simulink model "SFF_Simulator"  (R2024a)
settings: Solver=FixedStepAuto  StartTime=0.0  StopTime=tf  FixedStep=step_modelo  RelTol=1e-3
values from neighbouring files (symbols this model uses):
  AttKd_x = inp(4,2).Var2    [SFF_Simulator_Entradas.m]
  AttKd_y = inp(5,2).Var2    [SFF_Simulator_Entradas.m]
  AttKd_z = inp(6,2).Var2    [SFF_Simulator_Entradas.m]
  AttKp_x = inp(1,2).Var2    [SFF_Simulator_Entradas.m]
  AttKp_y = inp(2,2).Var2    [SFF_Simulator_Entradas.m]
  AttKp_z = inp(3,2).Var2    [SFF_Simulator_Entradas.m]
  beta = inp(2,2).Var2    [SFF_Simulator_Entradas.m]
  cdgps = inp(1,2).Var2    [SFF_Simulator_Entradas.m]
  estrelas = inp(4,2).Var2    [SFF_Simulator_Entradas.m]
  estrelas_bias = inp(6,2).Var2    [SFF_Simulator_Entradas.m]
  estrelas_ruido = inp(5,2).Var2    [SFF_Simulator_Entradas.m]
  gps_bias = inp(3,2).Var2    [SFF_Simulator_Entradas.m]
  gps_ruido = inp(2,2).Var2    [SFF_Simulator_Entradas.m]
  m1 = inp(6,2).Var2    [SFF_Simulator_Entradas.m]
  magne = inp(10,2).Var2    [SFF_Simulator_Entradas.m]
  magne_bias = inp(12,2).Var2    [SFF_Simulator_Entradas.m]
  magne_ruido = inp(11,2).Var2    [SFF_Simulator_Entradas.m]
  man = inp(1,2).Var2    [SFF_Simulator_Entradas.m]
  OrbKd_x = inp(3,2).Var2    [SFF_Simulator_Entradas.m]
  OrbKd_y = inp(6,2).Var2    [SFF_Simulator_Entradas.m]
  OrbKd_z = inp(9,2).Var2    [SFF_Simulator_Entradas.m]
  OrbKi_x = inp(2,2).Var2    [SFF_Simulator_Entradas.m]
  OrbKi_y = inp(5,2).Var2    [SFF_Simulator_Entradas.m]
  OrbKi_z = inp(8,2).Var2    [SFF_Simulator_Entradas.m]
  OrbKp_x = inp(1,2).Var2    [SFF_Simulator_Entradas.m]
  OrbKp_y = inp(4,2).Var2    [SFF_Simulator_Entradas.m]
  OrbKp_z = inp(7,2).Var2    [SFF_Simulator_Entradas.m]
  propForcaAtivo = inp(1,2).Var2    [SFF_Simulator_Entradas.m]
  rodaAtivo = inp(1,2).Var2    [SFF_Simulator_Entradas.m]
  torqrodAtivo = inp(1,2).Var2    [SFF_Simulator_Entradas.m]
undefined symbols (not defined in the file or in its folder): IAU, WMM2020
libraries: dspsrcs4 x9, aerolibtransform2 x1, aerolibgravity2 x1
(part 1 of 2)
settings Model: PacingRate=1000  VariantFading=off  Creator=rodri  LastModifiedBy=rodri
settings ModelReferenceCC: ModelReferenceMinAlgLoopOccurrences=on
settings RTWCC: GPUComputeCapability=3.5

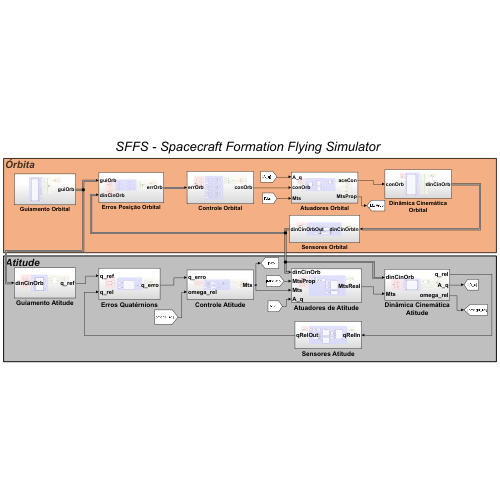
[thumbnail: Simulink's stored preview of the top-level diagram]
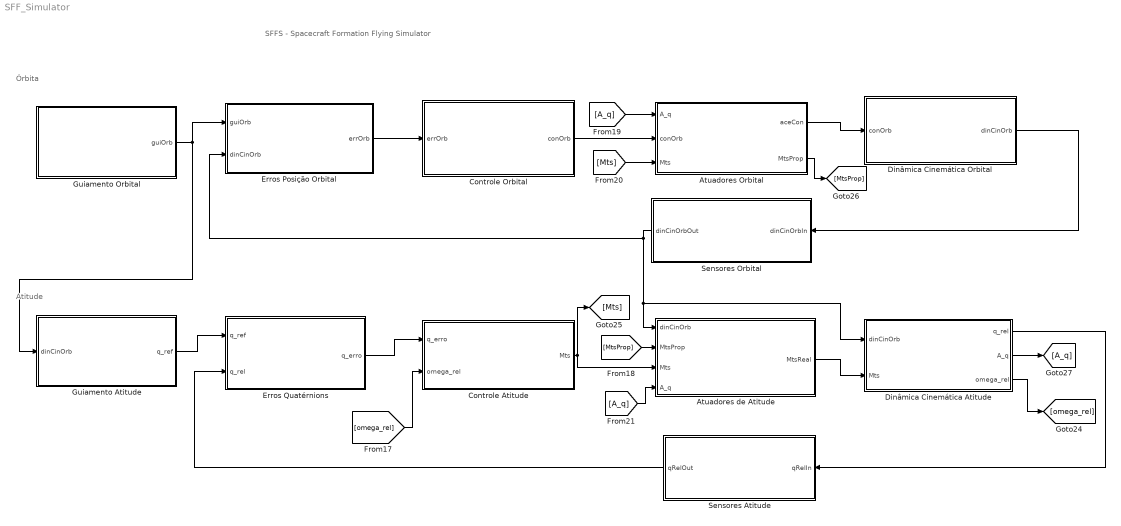
== system SFF_Simulator ==
  note: SFFS - Spacecraft Formation Flying Simulator
  note: Atitude
  note: Órbita
  Atuadores Orbital : Subsystem
  Atuadores de Atitude : Subsystem
  Controle Atitude : Subsystem
  Controle Orbital : Subsystem
  Dinâmica Cinemática Atitude : Subsystem
  Dinâmica Cinemática Orbital : Subsystem
  Erros Posição Orbital : Subsystem
  Erros Quatérnions : Subsystem
  Guiamento Atitude : Subsystem
  Guiamento Orbital : Subsystem
  Sensores Atitude : Subsystem
  Sensores Orbital : Subsystem
  wires:
  [omega_rel] -> Controle Atitude/2(omega_rel)
  Erros Quatérnions/1(q_erro) -> Controle Atitude/1(q_erro)
  Dinâmica Cinemática Atitude/2(A_q) -> [A_q]
  [A_q] -> Atuadores Orbital/1(A_q)
  Atuadores Orbital/1(aceCon) -> Dinâmica Cinemática Orbital/1(conOrb)
  Erros Posição Orbital/1(errOrb) -> Controle Orbital/1(errOrb)
  Dinâmica Cinemática Atitude/1(q_rel) -> Sensores Atitude/1(qRelIn)
  Guiamento Orbital/1(guiOrb) -> Guiamento Atitude/1(dinCinOrb), Erros Posição Orbital/1(guiOrb)
  Dinâmica Cinemática Atitude/3(omega_rel) -> [omega_rel]
  Guiamento Atitude/1(q_ref) -> Erros Quatérnions/1(q_ref)
  [MtsProp] -> Atuadores de Atitude/2(MtsProp)
  [Mts] -> Atuadores Orbital/3(Mts)
  [A_q] -> Atuadores de Atitude/4(A_q)
  Controle Atitude/1(Mts) -> Atuadores de Atitude/3(Mts), [Mts]
  Atuadores de Atitude/1(MtsReal) -> Dinâmica Cinemática Atitude/2(Mts)
  Atuadores Orbital/2(MtsProp) -> [MtsProp]
  Sensores Orbital/1(dinCinOrbOut) -> Dinâmica Cinemática Atitude/1(dinCinOrb), Atuadores de Atitude/1(dinCinOrb), Erros Posição Orbital/2(dinCinOrb)
  Controle Orbital/1(conOrb) -> Atuadores Orbital/2(conOrb)
  Sensores Atitude/1(qRelOut) -> Erros Quatérnions/2(q_rel)
  Dinâmica Cinemática Orbital/1(dinCinOrb) -> Sensores Orbital/1(dinCinOrbIn)

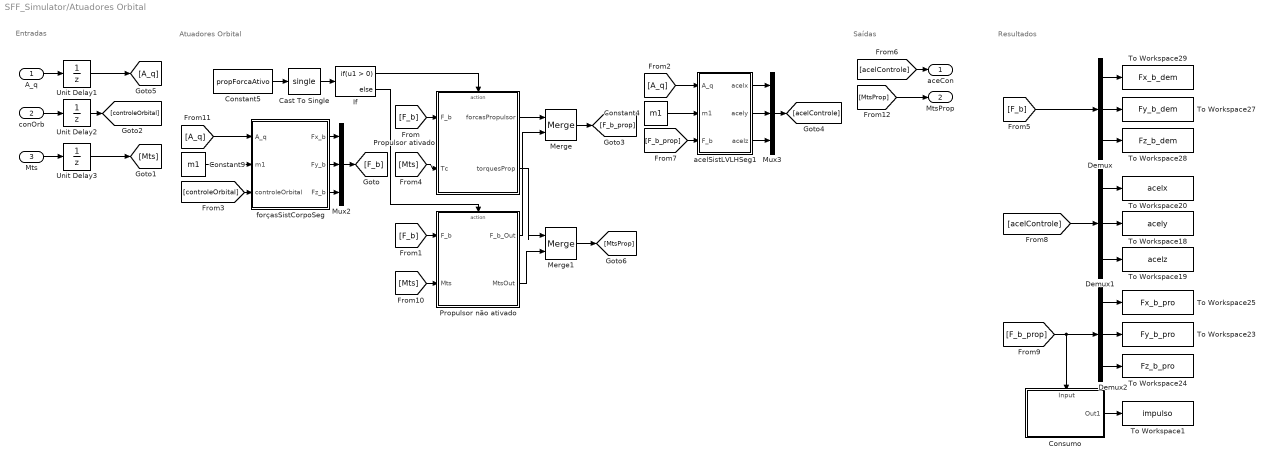
== system SFF_Simulator/Atuadores Orbital ==
  note: Resultados
  note: Entradas
  note: Saídas
  note: Atuadores Orbital
  A_q : Inport
  conOrb : Inport  Port=2
  Mts : Inport  Port=3
  Cast To Single : DataTypeConversion  OutDataTypeStr=single  SaturateOnIntegerOverflow=off  RndMeth=Floor
  Constant4 : Constant  Value=m1  SampleTime=-1
  Constant5 : Constant  Value=propForcaAtivo  SampleTime=-1
  Constant9 : Constant  Value=m1  SampleTime=-1
  Consumo : Subsystem
      settings: PortSchema="{\"entries\":[{\"content\":{\"sides\":[{\"content\":{},\"type\":\"ConnectorPlacement.EquallySpacedRectSide\",\"uuid\":\"7adfb598-cfd3-455e-a32c-0f282c9a4562\"},{\"content\":{\"connectorIds\":[\"Out1\"],\"side\":\"RIGHT\"},\"type\":\"ConnectorPlacement.EquallySpacedRectSide\",\"uuid\":\"983f0880-1b1d-4863-83b8-6f46272dfc63\"},{\"content\":{\"connectorIds\":[\"In1\"],\"side\":\"TOP\"},\"type\":\"ConnectorPlacement.EquallySpacedRectSide\",\"uuid\":\"1e4b7baa-07be-492c-ad2b-c1f0c72f4a8d\"}]},\"type\":\"ConnectorPlacement.EquallySpacedConnector\",\"uuid\":\"1ca021a5-bfd9-4f0e-bb93-1261a452b994\"}],\"packageUris\":[\"http://schema.mathworks.com/mf0/Connector/R2020b\"],\"version\":\"1.0\"}"
  Demux : Demux  Outputs=3
  Demux1 : Demux  Outputs=3
  Demux2 : Demux  Outputs=3
  If : If
  Merge : Merge
  Merge1 : Merge
  Mux2 : Mux  Inputs=3
  Mux3 : Mux  Inputs=3
  Propulsor ativado : Subsystem  TreatAsAtomicUnit=on
  Propulsor não ativado : Subsystem  TreatAsAtomicUnit=on
  To Workspace1 : ToWorkspace  VariableName=impulso  SampleTime=-1
      settings: Save2DSignal=2-D array (concatenate along first dimension)
  To Workspace18 : ToWorkspace  VariableName=acely  SampleTime=-1
      settings: Save2DSignal=2-D array (concatenate along first dimension)
  To Workspace19 : ToWorkspace  VariableName=acelz  SampleTime=-1
      settings: Save2DSignal=2-D array (concatenate along first dimension)
  To Workspace20 : ToWorkspace  VariableName=acelx  SampleTime=-1
      settings: Save2DSignal=2-D array (concatenate along first dimension)
  To Workspace23 : ToWorkspace  VariableName=Fy_b_pro  SampleTime=-1
      settings: Save2DSignal=2-D array (concatenate along first dimension)
  To Workspace24 : ToWorkspace  VariableName=Fz_b_pro  SampleTime=-1
      settings: Save2DSignal=2-D array (concatenate along first dimension)
  To Workspace25 : ToWorkspace  VariableName=Fx_b_pro  SampleTime=-1
      settings: Save2DSignal=2-D array (concatenate along first dimension)
  To Workspace27 : ToWorkspace  VariableName=Fy_b_dem  SampleTime=-1
      settings: Save2DSignal=2-D array (concatenate along first dimension)
  To Workspace28 : ToWorkspace  VariableName=Fz_b_dem  SampleTime=-1
      settings: Save2DSignal=2-D array (concatenate along first dimension)
  To Workspace29 : ToWorkspace  VariableName=Fx_b_dem  SampleTime=-1
      settings: Save2DSignal=2-D array (concatenate along first dimension)
  Unit Delay1 : UnitDelay  SampleTime=-1  HasFrameUpgradeWarning=on
  Unit Delay2 : UnitDelay  SampleTime=-1  HasFrameUpgradeWarning=on
  Unit Delay3 : UnitDelay  SampleTime=-1  HasFrameUpgradeWarning=on
  acelSistLVLHSeg1 : MATLAB Function  TreatAsAtomicUnit=on
  forçasSistCorpoSeg : MATLAB Function  TreatAsAtomicUnit=on
  aceCon : Outport
  MtsProp : Outport  Port=2
  wires:
  Demux1/3 -> To Workspace19/1
  Demux1/1 -> To Workspace20/1
  Demux1/2 -> To Workspace18/1
  [acelControle] -> Demux1/1
  Consumo/1(Out1) -> To Workspace1/1
  Demux/1 -> To Workspace29/1
  Demux/2 -> To Workspace27/1
  Demux/3 -> To Workspace28/1
  [F_b] -> Demux/1
  Demux2/1 -> To Workspace25/1
  [F_b_prop] -> Demux2/1, Consumo/1(Input)
  Demux2/2 -> To Workspace23/1
  Demux2/3 -> To Workspace24/1
  [A_q] -> acelSistLVLHSeg1/1(A_q)
  [acelControle] -> aceCon/1
  [F_b_prop] -> acelSistLVLHSeg1/3(F_b)
  [MtsProp] -> MtsProp/1
  Constant4/1 -> acelSistLVLHSeg1/2(m1)
  Propulsor ativado/2(torquesProp) -> Merge1/1
  Merge/1 -> [F_b_prop]
  forçasSistCorpoSeg/3(Fz_b) -> Mux2/3
  Unit Delay1/1 -> [A_q]
  Merge1/1 -> [MtsProp]
  forçasSistCorpoSeg/1(Fx_b) -> Mux2/1
  If/2 -> Propulsor não ativado/Action
  If/1 -> Propulsor ativado/Action
  Unit Delay2/1 -> [controleOrbital]
  [Mts] -> Propulsor não ativado/2(Mts)
  [A_q] -> forçasSistCorpoSeg/1(A_q)
  Constant9/1 -> forçasSistCorpoSeg/2(m1)
  [controleOrbital] -> forçasSistCorpoSeg/3(controleOrbital)
  [Mts] -> Propulsor ativado/2(Tc)
  acelSistLVLHSeg1/1(acelx) -> Mux3/1
  Mux3/1 -> [acelControle]
  acelSistLVLHSeg1/3(acelz) -> Mux3/3
  acelSistLVLHSeg1/2(acely) -> Mux3/2
  forçasSistCorpoSeg/2(Fy_b) -> Mux2/2
  Propulsor ativado/1(forcasPropulsor) -> Merge/1
  Cast To Single/1 -> If/1
  Mux2/1 -> [F_b]
  Mts/1 -> Unit Delay3/1
  [F_b] -> Propulsor não ativado/1(F_b)
  conOrb/1 -> Unit Delay2/1
  Propulsor não ativado/1(F_b_Out) -> Merge/2
  Unit Delay3/1 -> [Mts]
  Constant5/1 -> Cast To Single/1
  [F_b] -> Propulsor ativado/1(F_b)
  Propulsor não ativado/2(MtsOut) -> Merge1/2
  A_q/1 -> Unit Delay1/1

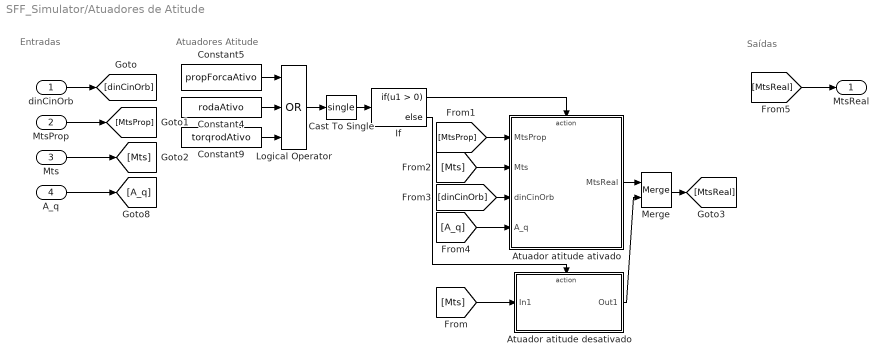
== system SFF_Simulator/Atuadores de Atitude ==
  note: Entradas
  note: Atuadores Atitude
  note: Saídas
  dinCinOrb : Inport
  MtsProp : Inport  Port=2
  Mts : Inport  Port=3
  A_q : Inport  Port=4
  Atuador atitude ativado : Subsystem  TreatAsAtomicUnit=on
  Atuador atitude desativado : Subsystem  TreatAsAtomicUnit=on
  Cast To Single : DataTypeConversion  OutDataTypeStr=single  SaturateOnIntegerOverflow=off  RndMeth=Floor
  Constant4 : Constant  Value=rodaAtivo  SampleTime=-1
  Constant5 : Constant  Value=propForcaAtivo  SampleTime=-1
  Constant9 : Constant  Value=torqrodAtivo  SampleTime=-1
  If : If
  Logical Operator : Logic  Operator=OR  Inputs=3  AllPortsSameDT=off  OutDataTypeStr=boolean
  Merge : Merge
  MtsReal : Outport
  wires:
  Mts/1 -> [Mts]
  dinCinOrb/1 -> [dinCinOrb]
  MtsProp/1 -> [MtsProp]
  Merge/1 -> [MtsReal]
  If/1 -> Atuador atitude ativado/Action
  If/2 -> Atuador atitude desativado/Action
  Atuador atitude ativado/1(MtsReal) -> Merge/1
  Atuador atitude desativado/1(Out1) -> Merge/2
  [Mts] -> Atuador atitude desativado/1(In1)
  [MtsProp] -> Atuador atitude ativado/1(MtsProp)
  [Mts] -> Atuador atitude ativado/2(Mts)
  [dinCinOrb] -> Atuador atitude ativado/3(dinCinOrb)
  [A_q] -> Atuador atitude ativado/4(A_q)
  A_q/1 -> [A_q]
  [MtsReal] -> MtsReal/1
  Constant5/1 -> Logical Operator/1
  Logical Operator/1 -> Cast To Single/1
  Cast To Single/1 -> If/1
  Constant4/1 -> Logical Operator/2
  Constant9/1 -> Logical Operator/3

== system SFF_Simulator/Controle Atitude ==
  note: Entradas
  note: Controle de Atitude
  note: Saídas
  note: Resultados
  q_erro : Inport
  omega_rel : Inport  Port=2
  Demux : Demux
  Demux1 : Demux  Outputs=3
  Demux3 : Demux  Outputs=3
  Gain1 : Gain  Gain=-1
  Kd1 : Gain  Gain=[AttKd_x AttKd_y AttKd_z]'
  Kp1 : Gain  Gain=[AttKp_x AttKp_y AttKp_z]'
  Mux : Mux  Inputs=3
  Sum3 : Sum  Inputs=|++
  Terminator : Terminator
  To Workspace24 : ToWorkspace  VariableName=Mts_x  SampleTime=-1
      settings: Save2DSignal=2-D array (concatenate along first dimension)
  To Workspace25 : ToWorkspace  VariableName=Mts_y  SampleTime=-1
      settings: Save2DSignal=2-D array (concatenate along first dimension)
  To Workspace26 : ToWorkspace  VariableName=Mts_z  SampleTime=-1
      settings: Save2DSignal=2-D array (concatenate along first dimension)
  Unit Delay : UnitDelay  SampleTime=-1  HasFrameUpgradeWarning=on
  Unit Delay1 : UnitDelay  SampleTime=-1  HasFrameUpgradeWarning=on
  Vector Concatenate1 : Concatenate  NumInputs=3  Mode=Multidimensional array
  Mts : Outport
  wires:
  [q_erro] -> Demux/1
  Mux/1 -> Kp1/1
  Demux/1 -> Mux/1
  Demux/2 -> Mux/2
  Demux/3 -> Mux/3
  Demux/4 -> Terminator/1
  [omega_rel] -> Kd1/1
  Kd1/1 -> Sum3/2
  Sum3/1 -> Demux1/1
  Demux1/1 -> Vector Concatenate1/1
  Demux1/2 -> Vector Concatenate1/2
  Demux1/3 -> Vector Concatenate1/3
  q_erro/1 -> Unit Delay/1
  omega_rel/1 -> Unit Delay1/1
  [Mts] -> Mts/1
  Vector Concatenate1/1 -> Gain1/1
  Gain1/1 -> [Mts]
  Kp1/1 -> Sum3/1
  Demux3/3 -> To Workspace26/1
  Demux3/2 -> To Workspace25/1
  Demux3/1 -> To Workspace24/1
  [Mts] -> Demux3/1
  Unit Delay/1 -> [q_erro]
  Unit Delay1/1 -> [omega_rel]

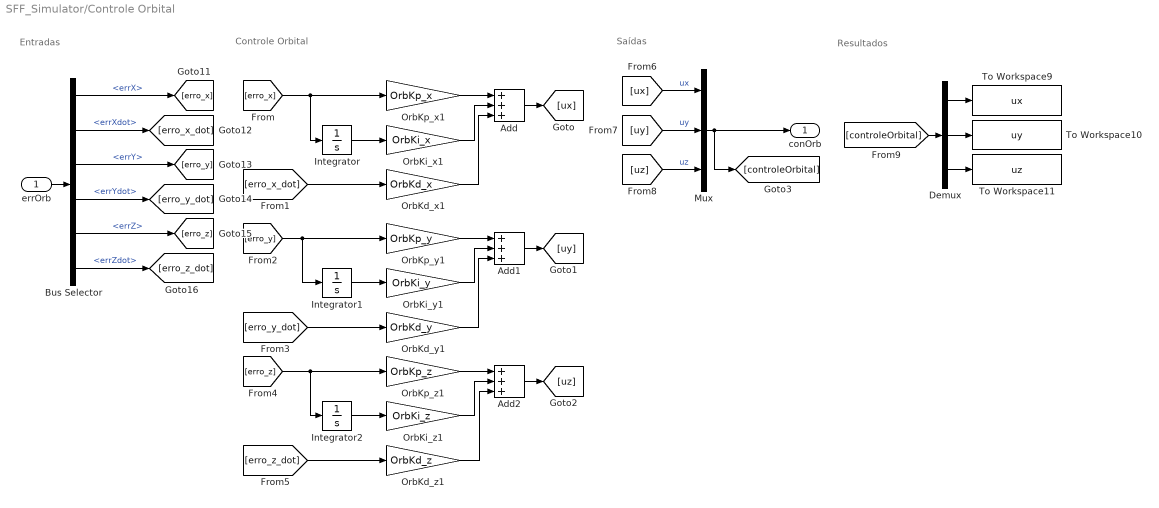
== system SFF_Simulator/Controle Orbital ==
  note: Entradas
  note: Controle Orbital
  note: Saídas
  note: Resultados
  errOrb : Inport
  Add : Sum  Inputs=+++
  Add1 : Sum  Inputs=+++
  Add2 : Sum  Inputs=+++
  Bus Selector : BusSelector  OutputSignals=errX,errXdot,errY,errYdot,errZ,errZdot
  Demux : Demux  Outputs=3
  Integrator : Integrator
  Integrator1 : Integrator
  Integrator2 : Integrator
  Mux : Mux  Inputs=3
  OrbKd_x1 : Gain  Gain=OrbKd_x
  OrbKd_y1 : Gain  Gain=OrbKd_y
  OrbKd_z1 : Gain  Gain=OrbKd_z
  OrbKi_x1 : Gain  Gain=OrbKi_x
  OrbKi_y1 : Gain  Gain=OrbKi_y
  OrbKi_z1 : Gain  Gain=OrbKi_z
  OrbKp_x1 : Gain  Gain=OrbKp_x
  OrbKp_y1 : Gain  Gain=OrbKp_y
  OrbKp_z1 : Gain  Gain=OrbKp_z
  To Workspace10 : ToWorkspace  VariableName=uy  SampleTime=-1
      settings: Save2DSignal=2-D array (concatenate along first dimension)
  To Workspace11 : ToWorkspace  VariableName=uz  SampleTime=-1
      settings: Save2DSignal=2-D array (concatenate along first dimension)
  To Workspace9 : ToWorkspace  VariableName=ux  SampleTime=-1
      settings: Save2DSignal=2-D array (concatenate along first dimension)
  conOrb : Outport
  wires:
  Add/1 -> [ux]
  Add1/1 -> [uy]
  Add2/1 -> [uz]
  Bus Selector/6 -> [erro_z_dot]  "<errZdot>"
  Bus Selector/4 -> [erro_y_dot]  "<errYdot>"
  Bus Selector/3 -> [erro_y]  "<errY>"
  Bus Selector/1 -> [erro_x]  "<errX>"
  Bus Selector/5 -> [erro_z]  "<errZ>"
  Bus Selector/2 -> [erro_x_dot]  "<errXdot>"
  errOrb/1 -> Bus Selector/1
  [ux] -> Mux/1  "ux"
  [uy] -> Mux/2  "uy"
  [uz] -> Mux/3  "uz"
  [erro_x_dot] -> OrbKd_x1/1
  Integrator1/1 -> OrbKi_y1/1
  Integrator2/1 -> OrbKi_z1/1
  [erro_y] -> OrbKp_y1/1, Integrator1/1
  OrbKi_z1/1 -> Add2/2
  OrbKi_x1/1 -> Add/2
  OrbKp_x1/1 -> Add/1
  OrbKd_x1/1 -> Add/3
  [erro_x] -> OrbKp_x1/1, Integrator/1
  OrbKi_y1/1 -> Add1/2
  OrbKp_y1/1 -> Add1/1
  Integrator/1 -> OrbKi_x1/1
  OrbKd_y1/1 -> Add1/3
  [erro_z_dot] -> OrbKd_z1/1
  OrbKd_z1/1 -> Add2/3
  [erro_y_dot] -> OrbKd_y1/1
  [erro_z] -> OrbKp_z1/1, Integrator2/1
  OrbKp_z1/1 -> Add2/1
  Mux/1 -> conOrb/1, [controleOrbital]
  Demux/3 -> To Workspace11/1
  [controleOrbital] -> Demux/1
  Demux/1 -> To Workspace9/1
  Demux/2 -> To Workspace10/1

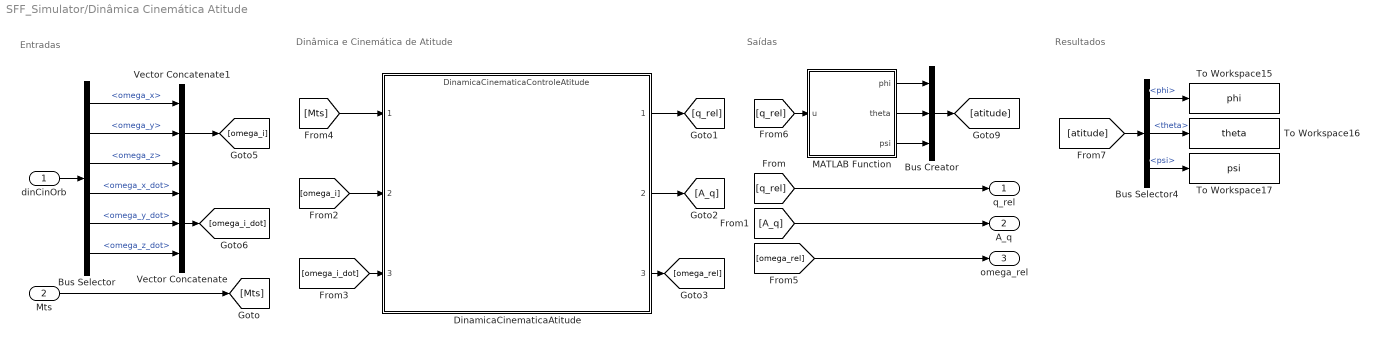
== system SFF_Simulator/Dinâmica Cinemática Atitude ==
  note: Dinâmica e Cinemática de Atitude
  note: Saídas
  note: Entradas
  note: Resultados
  dinCinOrb : Inport
  Mts : Inport  Port=2
  Bus Creator : BusCreator  Inputs=3
  Bus Selector : BusSelector  OutputSignals=omega_x,omega_y,omega_z,omega_x_dot,omega_y_dot,omega_z_dot
  Bus Selector4 : BusSelector  OutputSignals=phi,theta,psi
  DinamicaCinematicaAtitude : ModelReference  ModelNameDialog=DinamicaCinematicaControleAtitude  ModelReferenceVersion=3.15
  MATLAB Function : MATLAB Function  TreatAsAtomicUnit=on
  To Workspace15 : ToWorkspace  VariableName=phi  SampleTime=-1
      settings: Save2DSignal=2-D array (concatenate along first dimension)
  To Workspace16 : ToWorkspace  VariableName=theta  SampleTime=-1
      settings: Save2DSignal=2-D array (concatenate along first dimension)
  To Workspace17 : ToWorkspace  VariableName=psi  SampleTime=-1
      settings: Save2DSignal=2-D array (concatenate along first dimension)
  Vector Concatenate : Concatenate  NumInputs=3  Mode=Multidimensional array
  Vector Concatenate1 : Concatenate  NumInputs=3  Mode=Multidimensional array
  q_rel : Outport
  A_q : Outport  Port=2
  omega_rel : Outport  Port=3
  wires:
  DinamicaCinematicaAtitude/1 -> [q_rel]
  DinamicaCinematicaAtitude/2 -> [A_q]
  [q_rel] -> q_rel/1
  dinCinOrb/1 -> Bus Selector/1
  [omega_i] -> DinamicaCinematicaAtitude/2
  [omega_i_dot] -> DinamicaCinematicaAtitude/3
  [Mts] -> DinamicaCinematicaAtitude/1
  Bus Selector/1 -> Vector Concatenate1/1  "<omega_x>"
  Bus Selector/3 -> Vector Concatenate1/3  "<omega_z>"
  Bus Selector/2 -> Vector Concatenate1/2  "<omega_y>"
  Vector Concatenate1/1 -> [omega_i]
  Bus Selector/4 -> Vector Concatenate/1  "<omega_x_dot>"
  Bus Selector/5 -> Vector Concatenate/2  "<omega_y_dot>"
  Bus Selector/6 -> Vector Concatenate/3  "<omega_z_dot>"
  Vector Concatenate/1 -> [omega_i_dot]
  DinamicaCinematicaAtitude/3 -> [omega_rel]
  Mts/1 -> [Mts]
  [q_rel] -> MATLAB Function/1(u)
  MATLAB Function/1(phi) -> Bus Creator/1
  MATLAB Function/2(theta) -> Bus Creator/2
  MATLAB Function/3(psi) -> Bus Creator/3
  [A_q] -> A_q/1
  [omega_rel] -> omega_rel/1
  Bus Selector4/2 -> To Workspace16/1  "<theta>"
  Bus Selector4/1 -> To Workspace15/1  "<phi>"
  [atitude] -> Bus Selector4/1
  Bus Selector4/3 -> To Workspace17/1  "<psi>"
  Bus Creator/1 -> [atitude]

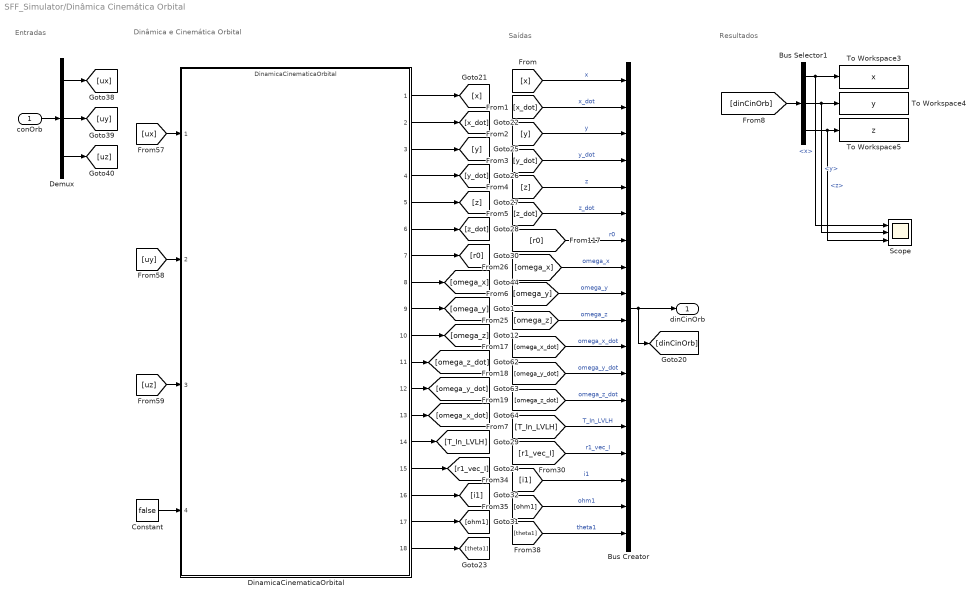
== system SFF_Simulator/Dinâmica Cinemática Orbital ==
  note: Entradas
  note: Saídas
  note: Dinâmica e Cinemática Orbital
  note: Resultados
  conOrb : Inport  OutDataTypeStr=double
  Bus Creator : BusCreator  Inputs=18
  Bus Selector1 : BusSelector  OutputSignals=x,y,z
  Constant : Constant  Value=false
  Demux : Demux  Outputs=3
  DinamicaCinematicaOrbital : ModelReference  ModelNameDialog=DinamicaCinematicaOrbital  ModelReferenceVersion=5.21
  Scope : Scope  NumInputPorts=3
  To Workspace3 : ToWorkspace  VariableName=x  SampleTime=-1
      settings: Save2DSignal=2-D array (concatenate along first dimension)
  To Workspace4 : ToWorkspace  VariableName=y  SampleTime=-1
      settings: Save2DSignal=2-D array (concatenate along first dimension)
  To Workspace5 : ToWorkspace  VariableName=z  SampleTime=-1
      settings: Save2DSignal=2-D array (concatenate along first dimension)
  dinCinOrb : Outport
  wires:
  conOrb/1 -> Demux/1
  Demux/1 -> [ux]
  Demux/2 -> [uy]
  Demux/3 -> [uz]
  [ux] -> DinamicaCinematicaOrbital/1
  [uy] -> DinamicaCinematicaOrbital/2
  [uz] -> DinamicaCinematicaOrbital/3
  Constant/1 -> DinamicaCinematicaOrbital/4
  Bus Creator/1 -> dinCinOrb/1, [dinCinOrb]
  Bus Selector1/1 -> To Workspace3/1, Scope/1  "<x>"
  Bus Selector1/2 -> To Workspace4/1, Scope/2  "<y>"
  Bus Selector1/3 -> Scope/3, To Workspace5/1  "<z>"
  [dinCinOrb] -> Bus Selector1/1
  DinamicaCinematicaOrbital/2 -> [x_dot]
  DinamicaCinematicaOrbital/5 -> [z]
  DinamicaCinematicaOrbital/4 -> [y_dot]
  DinamicaCinematicaOrbital/6 -> [z_dot]
  DinamicaCinematicaOrbital/7 -> [r0]
  DinamicaCinematicaOrbital/3 -> [y]
  DinamicaCinematicaOrbital/1 -> [x]
  DinamicaCinematicaOrbital/8 -> [omega_x]
  DinamicaCinematicaOrbital/10 -> [omega_z]
  DinamicaCinematicaOrbital/11 -> [omega_z_dot]
  DinamicaCinematicaOrbital/12 -> [omega_y_dot]
  DinamicaCinematicaOrbital/13 -> [omega_x_dot]
  DinamicaCinematicaOrbital/14 -> [T_In_LVLH]
  DinamicaCinematicaOrbital/15 -> [r1_vec_I]
  DinamicaCinematicaOrbital/16 -> [i1]
  DinamicaCinematicaOrbital/17 -> [ohm1]
  DinamicaCinematicaOrbital/18 -> [theta1]
  DinamicaCinematicaOrbital/9 -> [omega_y]
  [theta1] -> Bus Creator/18  "theta1"
  [ohm1] -> Bus Creator/17  "ohm1"
  [i1] -> Bus Creator/16  "i1"
  [r1_vec_I] -> Bus Creator/15  "r1_vec_I"
  [T_In_LVLH] -> Bus Creator/14  "T_In_LVLH"
  [omega_z_dot] -> Bus Creator/13  "omega_z_dot"
  [omega_y_dot] -> Bus Creator/12  "omega_y_dot"
  [omega_x_dot] -> Bus Creator/11  "omega_x_dot"
  [omega_z] -> Bus Creator/10  "omega_z"
  [omega_y] -> Bus Creator/9  "omega_y"
  [omega_x] -> Bus Creator/8  "omega_x"
  [r0] -> Bus Creator/7  "r0"
  [z_dot] -> Bus Creator/6  "z_dot"
  [z] -> Bus Creator/5  "z"
  [y_dot] -> Bus Creator/4  "y_dot"
  [y] -> Bus Creator/3  "y"
  [x_dot] -> Bus Creator/2  "x_dot"
  [x] -> Bus Creator/1  "x"

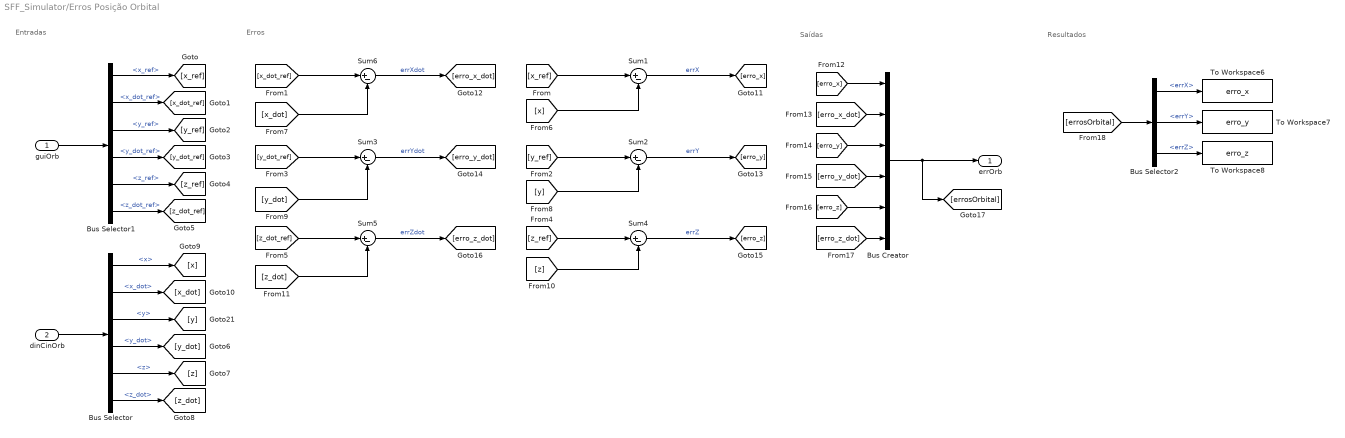
== system SFF_Simulator/Erros Posição Orbital ==
  note: Saídas
  note: Erros
  note: Entradas
  note: Resultados
  guiOrb : Inport
  dinCinOrb : Inport  Port=2
  Bus Creator : BusCreator  Inputs=6
  Bus Selector : BusSelector  OutputSignals=x,x_dot,y,y_dot,z,z_dot
  Bus Selector1 : BusSelector  OutputSignals=x_ref,x_dot_ref,y_ref,y_dot_ref,z_ref,z_dot_ref
  Bus Selector2 : BusSelector  OutputSignals=errX,errY,errZ
  Sum{1..6} (6 alike) : Sum  Inputs=|+-
  To Workspace6 : ToWorkspace  VariableName=erro_x  SampleTime=-1
      settings: Save2DSignal=2-D array (concatenate along first dimension)
  To Workspace7 : ToWorkspace  VariableName=erro_y  SampleTime=-1
      settings: Save2DSignal=2-D array (concatenate along first dimension)
  To Workspace8 : ToWorkspace  VariableName=erro_z  SampleTime=-1
      settings: Save2DSignal=2-D array (concatenate along first dimension)
  errOrb : Outport
  wires:
  [x] -> Sum1/2
  [x_dot] -> Sum6/2
  [x_dot_ref] -> Sum6/1
  [x_ref] -> Sum1/1
  Sum6/1 -> [erro_x_dot]  "errXdot"
  Sum1/1 -> [erro_x]  "errX"
  Sum3/1 -> [erro_y_dot]  "errYdot"
  Sum2/1 -> [erro_y]  "errY"
  [y] -> Sum2/2
  [y_dot] -> Sum3/2
  [y_ref] -> Sum2/1
  [y_dot_ref] -> Sum3/1
  Sum5/1 -> [erro_z_dot]  "errZdot"
  Sum4/1 -> [erro_z]  "errZ"
  [z_dot] -> Sum5/2
  [z_dot_ref] -> Sum5/1
  [z] -> Sum4/2
  [z_ref] -> Sum4/1
  Bus Selector1/4 -> [y_dot_ref]  "<y_dot_ref>"
  Bus Selector1/2 -> [x_dot_ref]  "<x_dot_ref>"
  guiOrb/1 -> Bus Selector1/1
  Bus Selector1/6 -> [z_dot_ref]  "<z_dot_ref>"
  Bus Selector1/3 -> [y_ref]  "<y_ref>"
  Bus Selector1/1 -> [x_ref]  "<x_ref>"
  Bus Selector1/5 -> [z_ref]  "<z_ref>"
  Bus Selector/1 -> [x]  "<x>"
  Bus Selector/4 -> [y_dot]  "<y_dot>"
  Bus Selector/3 -> [y]  "<y>"
  Bus Selector/6 -> [z_dot]  "<z_dot>"
  Bus Selector/5 -> [z]  "<z>"
  Bus Selector/2 -> [x_dot]  "<x_dot>"
  dinCinOrb/1 -> Bus Selector/1
  [erro_x] -> Bus Creator/1
  [erro_x_dot] -> Bus Creator/2
  [erro_y] -> Bus Creator/3
  [erro_y_dot] -> Bus Creator/4
  [erro_z] -> Bus Creator/5
  [erro_z_dot] -> Bus Creator/6
  Bus Selector2/2 -> To Workspace7/1  "<errY>"
  Bus Selector2/3 -> To Workspace8/1  "<errZ>"
  Bus Selector2/1 -> To Workspace6/1  "<errX>"
  [errosOrbital] -> Bus Selector2/1
  Bus Creator/1 -> [errosOrbital], errOrb/1

== system SFF_Simulator/Erros Quatérnions ==
  note: Erros
  note: Saídas
  note: Entradas
  q_ref : Inport
  q_rel : Inport  Port=2
  MATLAB Function4 : MATLAB Function  TreatAsAtomicUnit=on
  q_erro : Outport
  wires:
  [q_ref] -> MATLAB Function4/1(q_d)
  [q_rel] -> MATLAB Function4/2(q)
  MATLAB Function4/1(q_error) -> [q_erro]  "q_erro"
  [q_erro] -> q_erro/1
  q_rel/1 -> [q_rel]
  q_ref/1 -> [q_ref]

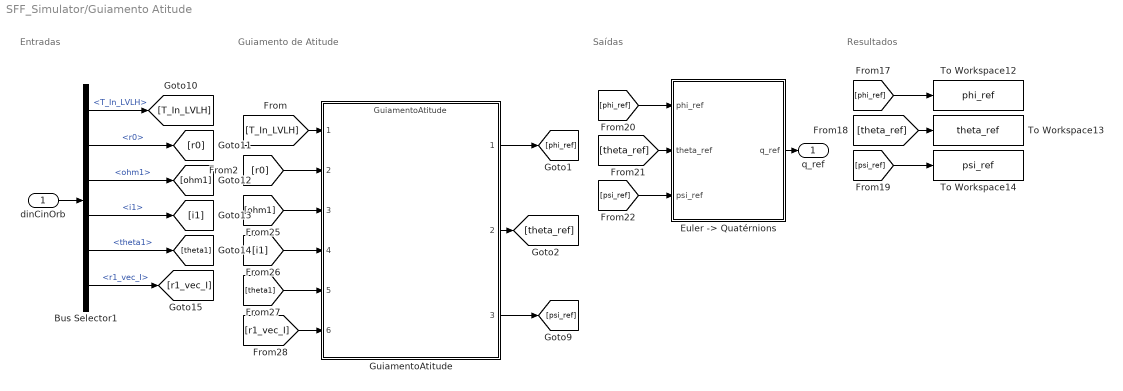
== system SFF_Simulator/Guiamento Atitude ==
  note: Entradas
  note: Guiamento de Atitude
  note: Saídas
  note: Resultados
  dinCinOrb : Inport
  Bus Selector1 : BusSelector  OutputSignals=T_In_LVLH,r0,ohm1,i1,theta1,r1_vec_I
  "Euler -> Quatérnions" : MATLAB Function  TreatAsAtomicUnit=on
  GuiamentoAtitude : ModelReference  ModelNameDialog=GuiamentoAtitude  ModelReferenceVersion=3.9
  To Workspace12 : ToWorkspace  VariableName=phi_ref  SampleTime=-1
      settings: Save2DSignal=2-D array (concatenate along first dimension)
  To Workspace13 : ToWorkspace  VariableName=theta_ref  SampleTime=-1
      settings: Save2DSignal=2-D array (concatenate along first dimension)
  To Workspace14 : ToWorkspace  VariableName=psi_ref  SampleTime=-1
      settings: Save2DSignal=2-D array (concatenate along first dimension)
  q_ref : Outport
  wires:
  dinCinOrb/1 -> Bus Selector1/1
  GuiamentoAtitude/2 -> [theta_ref]
  [r0] -> GuiamentoAtitude/2
  [ohm1] -> GuiamentoAtitude/3
  [theta1] -> GuiamentoAtitude/5
  GuiamentoAtitude/1 -> [phi_ref]
  GuiamentoAtitude/3 -> [psi_ref]
  [r1_vec_I] -> GuiamentoAtitude/6
  [i1] -> GuiamentoAtitude/4
  [T_In_LVLH] -> GuiamentoAtitude/1
  [theta_ref] -> To Workspace13/1
  [phi_ref] -> To Workspace12/1
  [phi_ref] -> "Euler -> Quatérnions"/1(phi_ref)
  [psi_ref] -> "Euler -> Quatérnions"/3(psi_ref)
  [psi_ref] -> To Workspace14/1
  [theta_ref] -> "Euler -> Quatérnions"/2(theta_ref)
  "Euler -> Quatérnions"/1(q_ref) -> q_ref/1
  Bus Selector1/3 -> [ohm1]  "<ohm1>"
  Bus Selector1/5 -> [theta1]  "<theta1>"
  Bus Selector1/2 -> [r0]  "<r0>"
  Bus Selector1/4 -> [i1]  "<i1>"
  Bus Selector1/1 -> [T_In_LVLH]  "<T_In_LVLH>"
  Bus Selector1/6 -> [r1_vec_I]  "<r1_vec_I>"

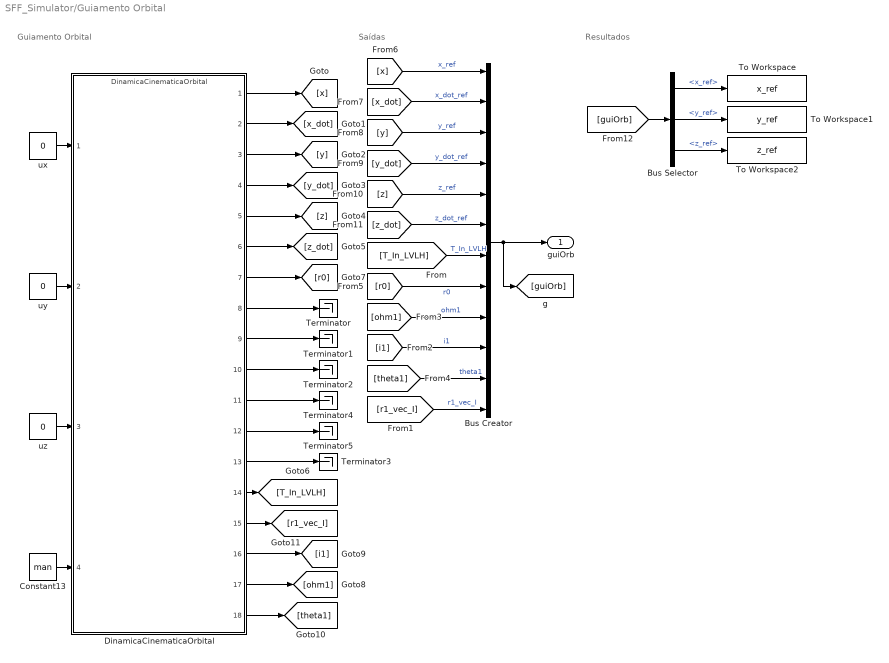
== system SFF_Simulator/Guiamento Orbital ==
  note: Saídas
  note: Guiamento Orbital
  note: Resultados
  Bus Creator : BusCreator  Inputs=12
  Bus Selector : BusSelector  OutputSignals=x_ref,y_ref,z_ref
  Constant13 : Constant  Value=man  OutDataTypeStr=boolean
  DinamicaCinematicaOrbital : ModelReference  ModelNameDialog=DinamicaCinematicaOrbital  ModelReferenceVersion=5.21
  Terminator{,1..5} (6 alike) : Terminator
  To Workspace : ToWorkspace  VariableName=x_ref  SampleTime=-1
      settings: Save2DSignal=2-D array (concatenate along first dimension)
  To Workspace1 : ToWorkspace  VariableName=y_ref  SampleTime=-1
      settings: Save2DSignal=2-D array (concatenate along first dimension)
  To Workspace2 : ToWorkspace  VariableName=z_ref  SampleTime=-1
      settings: Save2DSignal=2-D array (concatenate along first dimension)
  ux : Constant  Value=0
  uy : Constant  Value=0
  uz : Constant  Value=0
  guiOrb : Outport
  wires:
  [x] -> Bus Creator/1  "x_ref"
  [x_dot] -> Bus Creator/2  "x_dot_ref"
  [y] -> Bus Creator/3  "y_ref"
  [y_dot] -> Bus Creator/4  "y_dot_ref"
  [z] -> Bus Creator/5  "z_ref"
  [z_dot] -> Bus Creator/6  "z_dot_ref"
  Bus Creator/1 -> [guiOrb], guiOrb/1
  ux/1 -> DinamicaCinematicaOrbital/1
  uy/1 -> DinamicaCinematicaOrbital/2
  uz/1 -> DinamicaCinematicaOrbital/3
  Constant13/1 -> DinamicaCinematicaOrbital/4
  [r0] -> Bus Creator/8  "r0"
  [T_In_LVLH] -> Bus Creator/7  "T_In_LVLH"
  [ohm1] -> Bus Creator/9  "ohm1"
  [i1] -> Bus Creator/10  "i1"
  [theta1] -> Bus Creator/11  "theta1"
  [r1_vec_I] -> Bus Creator/12  "r1_vec_I"
  Bus Selector/3 -> To Workspace2/1  "<z_ref>"
  Bus Selector/2 -> To Workspace1/1  "<y_ref>"
  Bus Selector/1 -> To Workspace/1  "<x_ref>"
  [guiOrb] -> Bus Selector/1
  DinamicaCinematicaOrbital/1 -> [x]
  DinamicaCinematicaOrbital/2 -> [x_dot]
  DinamicaCinematicaOrbital/3 -> [y]
  DinamicaCinematicaOrbital/4 -> [y_dot]
  DinamicaCinematicaOrbital/5 -> [z]
  DinamicaCinematicaOrbital/6 -> [z_dot]
  DinamicaCinematicaOrbital/7 -> [r0]
  DinamicaCinematicaOrbital/8 -> Terminator/1
  DinamicaCinematicaOrbital/9 -> Terminator1/1
  DinamicaCinematicaOrbital/10 -> Terminator2/1
  DinamicaCinematicaOrbital/11 -> Terminator4/1
  DinamicaCinematicaOrbital/12 -> Terminator5/1
  DinamicaCinematicaOrbital/18 -> [theta1]
  DinamicaCinematicaOrbital/17 -> [ohm1]
  DinamicaCinematicaOrbital/16 -> [i1]
  DinamicaCinematicaOrbital/15 -> [r1_vec_I]
  DinamicaCinematicaOrbital/14 -> [T_In_LVLH]
  DinamicaCinematicaOrbital/13 -> Terminator3/1

== system SFF_Simulator/Sensores Atitude ==
  note: Entradas
  note: Sensor de Estrelas
  note: Saídas
  qRelIn : Inport
  Cast To Single : DataTypeConversion  OutDataTypeStr=single  SaturateOnIntegerOverflow=off  RndMeth=Floor
  Constant : Constant  Value=estrelas
  Demux : Demux  Outputs=3
  "Euler -> Quat" : MATLAB Function  TreatAsAtomicUnit=on
  If : If  IfExpression=u1 ~= 0
  Merge : Merge
  Mux1 : Mux  Inputs=3
  "Quat -> Euler" : MATLAB Function  TreatAsAtomicUnit=on
  Sensor ativado : Subsystem  TreatAsAtomicUnit=on
  Sensor desativado : Subsystem  TreatAsAtomicUnit=on
  qRelOut : Outport
  wires:
  Constant/1 -> Cast To Single/1
  Cast To Single/1 -> If/1
  If/1 -> Sensor ativado/Action
  If/2 -> Sensor desativado/Action
  Sensor desativado/1(atitudeOut) -> Merge/2
  Sensor ativado/1(atitudeOut) -> Merge/1
  "Quat -> Euler"/1(phi) -> Mux1/1
  "Quat -> Euler"/3(psi) -> Mux1/3
  "Quat -> Euler"/2(theta) -> Mux1/2
  Merge/1 -> Demux/1
  Demux/3 -> "Euler -> Quat"/3(psi_ref)
  Demux/2 -> "Euler -> Quat"/2(theta_ref)
  Demux/1 -> "Euler -> Quat"/1(phi_ref)
  Mux1/1 -> Sensor desativado/1(atitudeIn), Sensor ativado/1(atitudeIn)
  qRelIn/1 -> [q_rel]
  [q_rel] -> "Quat -> Euler"/1(u)
  [q_rel] -> "Euler -> Quat"/4(q_in)
  "Euler -> Quat"/1(q_ref) -> [q_relOut]
  [q_relOut] -> qRelOut/1

== system SFF_Simulator/Sensores Orbital ==
  note: Entradas
  note: Sensor GNSS/CDGNSS
  note: Saídas
  dinCinOrbIn : Inport
  Cast To Single : DataTypeConversion  OutDataTypeStr=single  SaturateOnIntegerOverflow=off  RndMeth=Floor
  Constant : Constant  Value=cdgps
  If : If  IfExpression=u1 ~= 0
  Merge : Merge
  Sensor ativado : Subsystem  TreatAsAtomicUnit=on
  Sensor desativado : Subsystem  TreatAsAtomicUnit=on
  dinCinOrbOut : Outport
  wires:
  Constant/1 -> Cast To Single/1
  Cast To Single/1 -> If/1
  If/1 -> Sensor ativado/Action
  If/2 -> Sensor desativado/Action
  Sensor desativado/1(dinCinOrbOut) -> Merge/2
  Sensor ativado/1(dinCinOrbOut) -> Merge/1
  dinCinOrbIn/1 -> [dinCinOrb]
  [dinCinOrb] -> Sensor ativado/1(dinCinOrbIn), Sensor desativado/1(dinCinOrbIn)
  Merge/1 -> [dinCinOrbSen]
  [dinCinOrbSen] -> dinCinOrbOut/1

== system SFF_Simulator/Atuadores Orbital/Consumo ==
  Input : Inport
  Abs1 : Abs  SaturateOnIntegerOverflow=off
  Abs2 : Abs  SaturateOnIntegerOverflow=off
  Abs3 : Abs  SaturateOnIntegerOverflow=off
  Add3 : Sum  Inputs=+++
  Demux : Demux  Outputs=3
  Integrator1 : Integrator
  Integrator2 : Integrator
  Integrator3 : Integrator
  Out1 : Outport  VectorParamsAs1DForOutWhenUnconnected=off
  wires:
  Demux/1 -> Abs3/1  "Fx"
  Integrator2/1 -> Add3/2
  Demux/2 -> Abs1/1  "Fy"
  Demux/3 -> Abs2/1  "Fz"
  Integrator3/1 -> Add3/3
  Add3/1 -> Out1/1
  Abs3/1 -> Integrator1/1
  Abs1/1 -> Integrator2/1
  Abs2/1 -> Integrator3/1
  Integrator1/1 -> Add3/1
  Input/1 -> Demux/1

== system SFF_Simulator/Atuadores Orbital/Propulsor ativado ==
  note: Entradas
  note: Propulsores
  note: Saídas
  F_b : Inport
  Tc : Inport  Port=2
  Action Port : ActionPort  ActionPortLabel=if(u1 > 0)
  AtuadorNaoLinear : ModelReference  ModelNameDialog=AtuadorNaoLinear  ModelReferenceVersion=3.54
  forcasPropulsor : Outport
  torquesProp : Outport  Port=2
  wires:
  AtuadorNaoLinear/2 -> [torquesProp]
  AtuadorNaoLinear/1 -> [forcasProp]
  Tc/1 -> [Tc]
  [Tc] -> AtuadorNaoLinear/2
  F_b/1 -> [F_b]
  [F_b] -> AtuadorNaoLinear/1
  [forcasProp] -> forcasPropulsor/1
  [torquesProp] -> torquesProp/1

== system SFF_Simulator/Atuadores Orbital/Propulsor não ativado ==
  F_b : Inport
  Mts : Inport  Port=2
  Action Port : ActionPort  ActionPortLabel=else
  F_b_Out : Outport
  MtsOut : Outport  Port=2
  wires:
  F_b/1 -> F_b_Out/1
  Mts/1 -> MtsOut/1

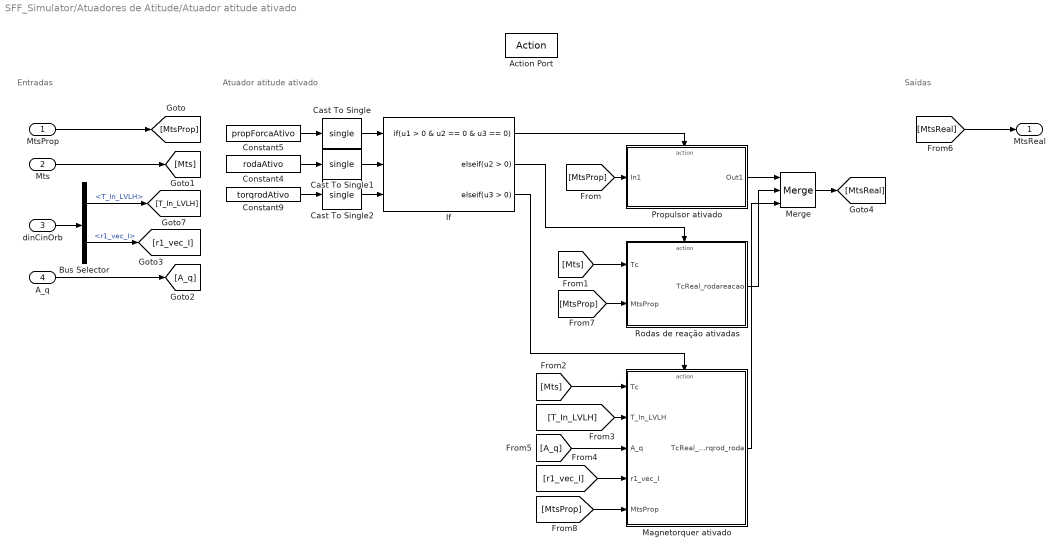
== system SFF_Simulator/Atuadores de Atitude/Atuador atitude ativado ==
  note: Entradas
  note: Atuador atitude ativado
  note: Saídas
  MtsProp : Inport
  Mts : Inport  Port=2
  dinCinOrb : Inport  Port=3
  A_q : Inport  Port=4
  Action Port : ActionPort  ActionPortLabel=if(u1 > 0)
  Bus Selector : BusSelector  OutputSignals=T_In_LVLH,r1_vec_I
  Cast To Single : DataTypeConversion  OutDataTypeStr=single  SaturateOnIntegerOverflow=off  RndMeth=Floor
  Cast To Single1 : DataTypeConversion  OutDataTypeStr=single  SaturateOnIntegerOverflow=off  RndMeth=Floor
  Cast To Single2 : DataTypeConversion  OutDataTypeStr=single  SaturateOnIntegerOverflow=off  RndMeth=Floor
  Constant4 : Constant  Value=rodaAtivo  SampleTime=-1
  Constant5 : Constant  Value=propForcaAtivo  SampleTime=-1
  Constant9 : Constant  Value=torqrodAtivo  SampleTime=-1
  If : If  NumInputs=3  IfExpression=u1 > 0 & u2 == 0 & u3 == 0  ElseIfExpressions=u2 > 0, u3 > 0  ShowElse=off
  Magnetorquer ativado : Subsystem  TreatAsAtomicUnit=on
  Merge : Merge  Inputs=3
  Propulsor ativado : Subsystem  TreatAsAtomicUnit=on
  Rodas de reação ativadas : Subsystem  TreatAsAtomicUnit=on
  MtsReal : Outport
  wires:
  Bus Selector/2 -> [r1_vec_I]  "<r1_vec_I>"
  Bus Selector/1 -> [T_In_LVLH]  "<T_In_LVLH>"
  dinCinOrb/1 -> Bus Selector/1
  If/1 -> Propulsor ativado/Action
  Propulsor ativado/1(Out1) -> Merge/1
  Rodas de reação ativadas/1(TcReal_rodareacao) -> Merge/2
  Magnetorquer ativado/1(TcReal_torqrod_roda) -> Merge/3
  If/3 -> Magnetorquer ativado/Action
  MtsProp/1 -> [MtsProp]
  Mts/1 -> [Mts]
  A_q/1 -> [A_q]
  Merge/1 -> [MtsReal]
  [MtsReal] -> MtsReal/1
  Constant9/1 -> Cast To Single2/1
  Cast To Single1/1 -> If/2
  Cast To Single2/1 -> If/3
  Constant4/1 -> Cast To Single1/1
  Cast To Single/1 -> If/1
  Constant5/1 -> Cast To Single/1
  [MtsProp] -> Propulsor ativado/1(In1)
  [Mts] -> Rodas de reação ativadas/1(Tc)
  If/2 -> Rodas de reação ativadas/Action
  [MtsProp] -> Rodas de reação ativadas/2(MtsProp)
  [A_q] -> Magnetorquer ativado/3(A_q)
  [T_In_LVLH] -> Magnetorquer ativado/2(T_In_LVLH)
  [r1_vec_I] -> Magnetorquer ativado/4(r1_vec_I)
  [Mts] -> Magnetorquer ativado/1(Tc)
  [MtsProp] -> Magnetorquer ativado/5(MtsProp)

== system SFF_Simulator/Atuadores de Atitude/Atuador atitude desativado ==
  In1 : Inport
  Action Port : ActionPort  ActionPortLabel=else
  Out1 : Outport
  wires:
  In1/1 -> Out1/1

== system SFF_Simulator/Sensores Atitude/Sensor ativado ==
  atitudeIn : Inport
  Action Port : ActionPort  ActionPortLabel=if(u1 ~= 0)
  Demux : Demux  Outputs=3
  Mux : Mux  Inputs=3
  estrelasSensor_phi : Subsystem
  estrelasSensor_psi : Subsystem
  estrelasSensor_theta : Subsystem
  atitudeOut : Outport
  wires:
  Demux/3 -> estrelasSensor_psi/1(In1)
  Demux/2 -> estrelasSensor_theta/1(In1)
  Demux/1 -> estrelasSensor_phi/1(phiIn)
  atitudeIn/1 -> Demux/1
  estrelasSensor_phi/1(phiOut) -> Mux/1
  estrelasSensor_theta/1(Out1) -> Mux/2
  estrelasSensor_psi/1(Out1) -> Mux/3
  Mux/1 -> atitudeOut/1

== system SFF_Simulator/Sensores Atitude/Sensor desativado ==
  atitudeIn : Inport
  Action Port : ActionPort  ActionPortLabel=else
  atitudeOut : Outport
  wires:
  atitudeIn/1 -> atitudeOut/1

== system SFF_Simulator/Sensores Orbital/Sensor ativado ==
  dinCinOrbIn : Inport
  Action Port : ActionPort  ActionPortLabel=if(u1 ~= 0)
  Bus Creator : BusCreator  Inputs=18
  Bus Selector : BusSelector  OutputSignals=x,y,z
  Bus Selector1 : BusSelector  OutputSignals=x_dot,y_dot,z_dot,r0,omega_x,omega_y,omega_z,omega_x_dot,omega_y_dot,omega_z_dot,T_In_LVLH,r1_vec_I,i1,ohm1,theta1
  GPSsensor : Subsystem
  GPSsensor1 : Subsystem
  GPSsensor2 : Subsystem
  dinCinOrbOut : Outport
  wires:
  Bus Selector/3 -> GPSsensor2/1(In1)  "<z>"
  Bus Selector/2 -> GPSsensor1/1(In1)  "<y>"
  Bus Selector/1 -> GPSsensor/1(In1)  "<x>"
  dinCinOrbIn/1 -> Bus Selector/1, Bus Selector1/1
  Bus Creator/1 -> dinCinOrbOut/1
  Bus Selector1/4 -> Bus Creator/7  "<r0>"
  Bus Selector1/5 -> Bus Creator/8  "<omega_x>"
  Bus Selector1/6 -> Bus Creator/9  "<omega_y>"
  Bus Selector1/7 -> Bus Creator/10  "<omega_z>"
  Bus Selector1/8 -> Bus Creator/11  "<omega_x_dot>"
  Bus Selector1/9 -> Bus Creator/12  "<omega_y_dot>"
  Bus Selector1/10 -> Bus Creator/13  "<omega_z_dot>"
  Bus Selector1/11 -> Bus Creator/14  "<T_In_LVLH>"
  Bus Selector1/12 -> Bus Creator/15  "<r1_vec_I>"
  Bus Selector1/13 -> Bus Creator/16  "<i1>"
  Bus Selector1/14 -> Bus Creator/17  "<ohm1>"
  Bus Selector1/15 -> Bus Creator/18  "<theta1>"
  GPSsensor2/1(Out1) -> Bus Creator/5  "z"
  GPSsensor1/1(Out1) -> Bus Creator/3  "y"
  GPSsensor/1(Out1) -> Bus Creator/1  "x"
  Bus Selector1/1 -> Bus Creator/2  "<x_dot>"
  Bus Selector1/2 -> Bus Creator/4  "<y_dot>"
  Bus Selector1/3 -> Bus Creator/6  "<z_dot>"

== system SFF_Simulator/Sensores Orbital/Sensor desativado ==
  dinCinOrbIn : Inport
  Action Port : ActionPort  ActionPortLabel=else
  dinCinOrbOut : Outport
  wires:
  dinCinOrbIn/1 -> dinCinOrbOut/1

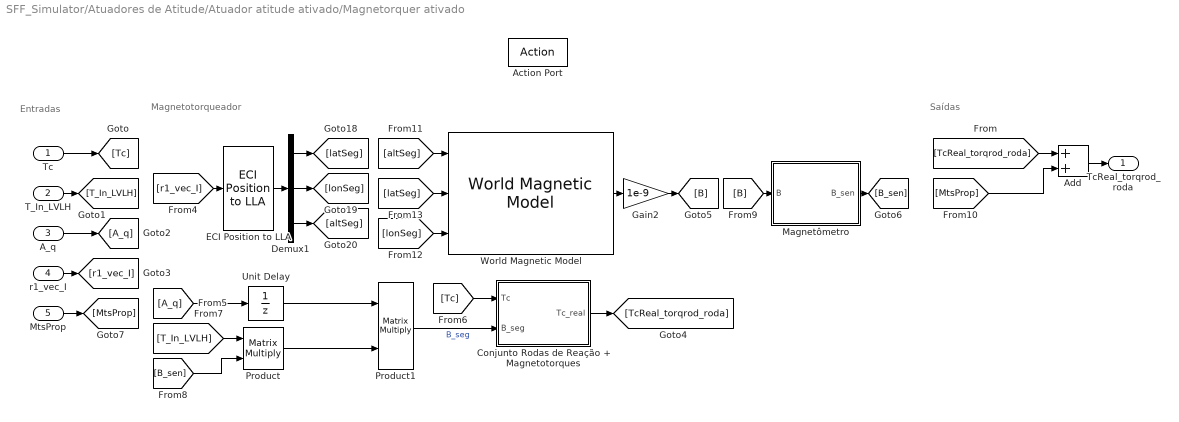
== system SFF_Simulator/Atuadores de Atitude/Atuador atitude ativado/Magnetorquer ativado ==
  note: Magnetotorqueador
  note: Saídas
  note: Entradas
  Tc : Inport
  T_In_LVLH : Inport  Port=2
  A_q : Inport  Port=3
  r1_vec_I : Inport  Port=4
  MtsProp : Inport  Port=5
  Action Port : ActionPort  ActionPortLabel=elseif( u3 > 0)
  Add : Sum
  Conjunto Rodas de Reação + Magnetotorques : Subsystem
  Demux1 : Demux  Outputs=3
  ECI Position to LLA : aerolibtransform2/ECI Position to LLA  red=IAU-2000/2006  year=2013  month=January  day=1  hour=0  min=0  sec=0  deltaT=None  errorflag=Error  extraparamflag=off  eunits=Metric (MKS)  earthmodel=WGS84  flat=1/298.257223563  eqradius=6378137
      settings: AttributesFormatString=%<red>
  Gain2 : Gain  Gain=1e-9
  Magnetômetro : Subsystem
  Product : Product  Multiplication=Matrix(*)
  Product1 : Product  Multiplication=Matrix(*)
  Unit Delay : UnitDelay  SampleTime=-1  HasFrameUpgradeWarning=on
  World Magnetic Model : aerolibgravity2/World Magnetic Model  model=WMM2020 (2020-2025)  customFile='WMM2020.COF'  units=Metric (MKS)  time_in=off  month=January  day=1  year=2024  action=Error  h_out=off  dec_out=off  inc_out=off  ti_out=off
  TcReal_torqrod_roda : Outport
  wires:
  Demux1/2 -> [lonSeg]
  Product/1 -> Product1/2
  Demux1/1 -> [latSeg]
  Demux1/3 -> [altSeg]
  Product1/1 -> Conjunto Rodas de Reação + Magnetotorques/2(B_seg)  "B_seg"
  Unit Delay/1 -> Product1/1
  [Tc] -> Conjunto Rodas de Reação + Magnetotorques/1(Tc)
  [A_q] -> Unit Delay/1
  [T_In_LVLH] -> Product/1
  Conjunto Rodas de Reação + Magnetotorques/1(Tc_real) -> [TcReal_torqrod_roda]
  Magnetômetro/1(B_sen) -> [B_sen]
  [B] -> Magnetômetro/1(B)
  Gain2/1 -> [B]
  [B_sen] -> Product/2
  [r1_vec_I] -> ECI Position to LLA/1
  ECI Position to LLA/1 -> Demux1/1
  [TcReal_torqrod_roda] -> Add/1
  [MtsProp] -> Add/2
  Add/1 -> TcReal_torqrod_roda/1
  T_In_LVLH/1 -> [T_In_LVLH]
  r1_vec_I/1 -> [r1_vec_I]
  MtsProp/1 -> [MtsProp]
  A_q/1 -> [A_q]
  Tc/1 -> [Tc]
  World Magnetic Model/1 -> Gain2/1
  [lonSeg] -> World Magnetic Model/3
  [latSeg] -> World Magnetic Model/2
  [altSeg] -> World Magnetic Model/1

== system SFF_Simulator/Atuadores de Atitude/Atuador atitude ativado/Propulsor ativado ==
  In1 : Inport
  Action Port : ActionPort  ActionPortLabel=if(u1 > 0 & u2 == 0 & u3 == 0)
  Out1 : Outport
  wires:
  In1/1 -> Out1/1

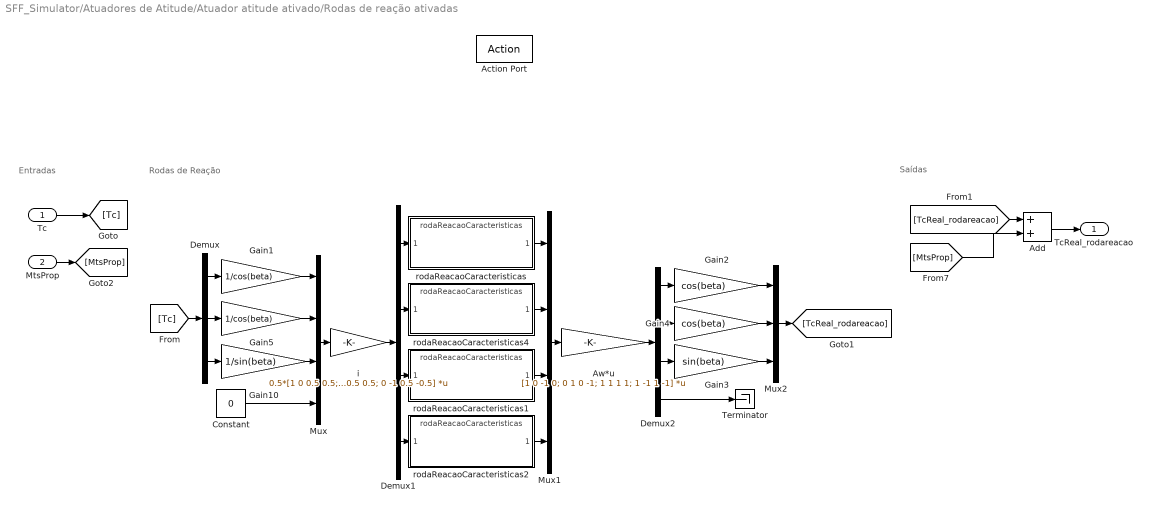
== system SFF_Simulator/Atuadores de Atitude/Atuador atitude ativado/Rodas de reação ativadas ==
  note: Rodas de Reação
  note: Entradas
  note: Saídas
  Tc : Inport
  MtsProp : Inport  Port=2
  Action Port : ActionPort  ActionPortLabel=elseif(u2 > 0)
  Add : Sum
  Aw*u : Gain  Gain=[1 0 -1 0; 0 1 0 -1; 1 1 1 1; 1 -1 1 -1]  Multiplication=Matrix(K*u)
  Constant : Constant  Value=0  SampleTime=-1
  Demux : Demux  Outputs=3
  Demux1 : Demux
  Demux2 : Demux
  Gain1 : Gain  Gain=1/cos(beta)
  Gain10 : Gain  Gain=1/sin(beta)
  Gain2 : Gain  Gain=cos(beta)
  Gain3 : Gain  Gain=sin(beta)
  Gain4 : Gain  Gain=cos(beta)
  Gain5 : Gain  Gain=1/cos(beta)
  Mux : Mux
  Mux1 : Mux
  Mux2 : Mux  Inputs=3
  Terminator : Terminator
  i : Gain  Gain=0.5*[1 0 0.5 0.5;0 1 0.5 -0.5; -1 0 0.5 0.5; 0 -1 0.5 -0.5]  Multiplication=Matrix(K*u)
  rodaReacaoCaracteristicas{,1..2,4} (4 alike) : ModelReference  ModelNameDialog=rodaReacaoCaracteristicas  ModelReferenceVersion=3.129
  TcReal_rodareacao : Outport
  wires:
  Mux2/1 -> [TcReal_rodareacao]
  rodaReacaoCaracteristicas2/1 -> Mux1/4
  Constant/1 -> Mux/4
  Mux/1 -> i/1
  Gain2/1 -> Mux2/1
  Demux2/1 -> Gain2/1
  Gain1/1 -> Mux/1
  Gain4/1 -> Mux2/2
  Demux2/4 -> Terminator/1
  Gain3/1 -> Mux2/3
  Gain10/1 -> Mux/3
  Mux1/1 -> Aw*u/1
  i/1 -> Demux1/1
  Demux/2 -> Gain5/1
  Demux2/3 -> Gain3/1
  rodaReacaoCaracteristicas1/1 -> Mux1/3
  Aw*u/1 -> Demux2/1
  Gain5/1 -> Mux/2
  rodaReacaoCaracteristicas/1 -> Mux1/1
  Demux/3 -> Gain10/1
  Demux/1 -> Gain1/1
  rodaReacaoCaracteristicas4/1 -> Mux1/2
  Demux2/2 -> Gain4/1
  Tc/1 -> [Tc]
  [Tc] -> Demux/1
  Demux1/4 -> rodaReacaoCaracteristicas2/1
  Demux1/3 -> rodaReacaoCaracteristicas1/1
  Demux1/2 -> rodaReacaoCaracteristicas4/1
  Demux1/1 -> rodaReacaoCaracteristicas/1
  [TcReal_rodareacao] -> Add/1
  [MtsProp] -> Add/2
  Add/1 -> TcReal_rodareacao/1
  MtsProp/1 -> [MtsProp]

== system SFF_Simulator/Sensores Atitude/Sensor ativado/estrelasSensor_phi ==
  phiIn : Inport
  Add1 : Sum
  Add2 : Sum
  Ruído : dspsrcs4/Random Source  SrcType=Uniform  MinVal=-estrelas_ruido  MaxVal=estrelas_ruido  MeanVal=0  VarVal=1  RepMode=Not repeatable  rawSeed=1  IsInherit=off  SampTime=step_modelo  SampFrame=1  OutComplex=Real  DataType=double  SimulateUsing=Code generation
  Viés : Constant  Value=estrelas_bias
  phiOut : Outport
  wires:
  Ruído/1 -> Add2/1
  phiIn/1 -> Add1/2
  Viés/1 -> Add1/1
  Add1/1 -> Add2/2
  Add2/1 -> phiOut/1

== system SFF_Simulator/Sensores Atitude/Sensor ativado/estrelasSensor_psi ==
  In1 : Inport
  Add1 : Sum
  Add2 : Sum
  Constant : Constant  Value=estrelas_bias
  Random Source1 : dspsrcs4/Random Source  SrcType=Uniform  MinVal=-estrelas_ruido  MaxVal=estrelas_ruido  MeanVal=0  VarVal=1  RepMode=Not repeatable  rawSeed=1  IsInherit=off  SampTime=step_modelo  SampFrame=1  OutComplex=Real  DataType=double  SimulateUsing=Code generation
  Out1 : Outport
  wires:
  Random Source1/1 -> Add2/1
  Constant/1 -> Add1/1
  Add2/1 -> Out1/1
  In1/1 -> Add1/2
  Add1/1 -> Add2/2

== system SFF_Simulator/Sensores Atitude/Sensor ativado/estrelasSensor_theta ==
  In1 : Inport
  Add1 : Sum
  Add2 : Sum
  Constant : Constant  Value=estrelas_bias
  Random Source1 : dspsrcs4/Random Source  SrcType=Uniform  MinVal=-estrelas_ruido  MaxVal=estrelas_ruido  MeanVal=0  VarVal=1  RepMode=Not repeatable  rawSeed=1  IsInherit=off  SampTime=step_modelo  SampFrame=1  OutComplex=Real  DataType=double  SimulateUsing=Code generation
  Out1 : Outport
  wires:
  Random Source1/1 -> Add2/1
  Constant/1 -> Add1/1
  Add2/1 -> Out1/1
  In1/1 -> Add1/2
  Add1/1 -> Add2/2

== system SFF_Simulator/Sensores Orbital/Sensor ativado/GPSsensor ==
  In1 : Inport
  Add1 : Sum
  Add2 : Sum
  Constant : Constant  Value=gps_bias
  Random Source1 : dspsrcs4/Random Source  SrcType=Uniform  MinVal=-gps_ruido  MaxVal=gps_ruido  MeanVal=0  VarVal=1  RepMode=Not repeatable  rawSeed=1  IsInherit=off  SampTime=step_modelo  SampFrame=1  OutComplex=Real  DataType=double  SimulateUsing=Code generation
  Out1 : Outport
  wires:
  Random Source1/1 -> Add2/1
  In1/1 -> Add1/2
  Constant/1 -> Add1/1
  Add1/1 -> Add2/2
  Add2/1 -> Out1/1

== system SFF_Simulator/Sensores Orbital/Sensor ativado/GPSsensor1 ==
  In1 : Inport
  Add1 : Sum
  Add2 : Sum
  Constant : Constant  Value=gps_bias
  Random Source1 : dspsrcs4/Random Source  SrcType=Uniform  MinVal=-gps_ruido  MaxVal=gps_ruido  MeanVal=0  VarVal=1  RepMode=Not repeatable  rawSeed=1  IsInherit=off  SampTime=step_modelo  SampFrame=1  OutComplex=Real  DataType=double  SimulateUsing=Code generation
  Out1 : Outport
  wires:
  Random Source1/1 -> Add2/1
  Constant/1 -> Add1/1
  Add1/1 -> Add2/2
  In1/1 -> Add1/2
  Add2/1 -> Out1/1

== system SFF_Simulator/Sensores Orbital/Sensor ativado/GPSsensor2 ==
  In1 : Inport
  Add1 : Sum
  Add2 : Sum
  Constant : Constant  Value=gps_bias
  Random Source1 : dspsrcs4/Random Source  SrcType=Uniform  MinVal=-gps_ruido  MaxVal=gps_ruido  MeanVal=0  VarVal=1  RepMode=Not repeatable  rawSeed=1  IsInherit=off  SampTime=step_modelo  SampFrame=1  OutComplex=Real  DataType=double  SimulateUsing=Code generation
  Out1 : Outport
  wires:
  Random Source1/1 -> Add2/1
  Constant/1 -> Add1/1
  Add1/1 -> Add2/2
  In1/1 -> Add1/2
  Add2/1 -> Out1/1

== system SFF_Simulator/Atuadores de Atitude/Atuador atitude ativado/Magnetorquer ativado/Conjunto Rodas de Reação + Magnetotorques ==
  note: Entradas
  note: Saídas
  note: Conjunto Rodas de Reação + Magnetotorqueadores
  Tc : Inport
  B_seg : Inport  Port=2
  B_matriz : MATLAB Function  TreatAsAtomicUnit=on
  Demux1 : Demux  Outputs=3
  Gain1 : Gain  Gain=-1
  Gain3 : Gain  Gain=-1
  Inv_B_matriz : MATLAB Function  TreatAsAtomicUnit=on
  MatrixMultiply : Product  Multiplication=Matrix(*)
  MatrixMultiply1 : Product  Multiplication=Matrix(*)
  Model : ModelReference  ModelNameDialog=rodaReacaoCaracteristicas.slx  ModelReferenceVersion=3.129
  Mux : Mux  Inputs=3
  magnetorquerCaracteristicas : ModelReference  ModelNameDialog=magnetorquerCaracteristicas  ModelReferenceVersion=3.127
  magnetorquerCaracteristicas1 : ModelReference  ModelNameDialog=magnetorquerCaracteristicas  ModelReferenceVersion=3.127
  Tc_real : Outport  VectorParamsAs1DForOutWhenUnconnected=off
  wires:
  B_matriz/1(y) -> MatrixMultiply1/1
  MatrixMultiply/1 -> Demux1/1
  Demux1/2 -> Gain1/1  "hwy_dot"
  Demux1/3 -> magnetorquerCaracteristicas1/1  "Mz"
  Mux/1 -> MatrixMultiply1/2
  Gain1/1 -> Model/1
  Model/1 -> Gain3/1
  Gain3/1 -> Mux/2
  Inv_B_matriz/1(y) -> MatrixMultiply/1
  Demux1/1 -> magnetorquerCaracteristicas/1  "Mx"
  magnetorquerCaracteristicas/1 -> Mux/1
  magnetorquerCaracteristicas1/1 -> Mux/3
  Tc/1 -> [Tc]
  [Tc] -> MatrixMultiply/2
  B_seg/1 -> [B_seg]
  [B_seg] -> Inv_B_matriz/1(B_seg), B_matriz/1(B_seg)
  MatrixMultiply1/1 -> [Tc_real]
  [Tc_real] -> Tc_real/1

== system SFF_Simulator/Atuadores de Atitude/Atuador atitude ativado/Magnetorquer ativado/Magnetômetro ==
  B : Inport
  Cast To Single : DataTypeConversion  OutDataTypeStr=single  SaturateOnIntegerOverflow=off  RndMeth=Floor
  Constant : Constant  Value=magne
  If : If  IfExpression=u1 ~= 0
  If Action Subsystem : Subsystem  TreatAsAtomicUnit=on
  If Action Subsystem1 : Subsystem  TreatAsAtomicUnit=on
  Merge : Merge
  B_sen : Outport
  wires:
  Cast To Single/1 -> If/1
  If/2 -> If Action Subsystem1/Action
  If Action Subsystem/1(atitudeSen) -> Merge/1
  If/1 -> If Action Subsystem/Action
  Merge/1 -> B_sen/1
  Constant/1 -> Cast To Single/1
  If Action Subsystem1/1(atitudeSen) -> Merge/2
  B/1 -> If Action Subsystem/1(atitude), If Action Subsystem1/1(atitude)

== system SFF_Simulator/Atuadores de Atitude/Atuador atitude ativado/Magnetorquer ativado/Magnetômetro/If Action Subsystem ==
  atitude : Inport
  Action Port : ActionPort  ActionPortLabel=if(u1 ~= 0)
  Demux : Demux  Outputs=3
  Mux : Mux  Inputs=3
  magneSensor : Subsystem
  magneSensor1 : Subsystem
  magneSensor2 : Subsystem
  atitudeSen : Outport
  wires:
  Demux/3 -> magneSensor2/1(In1)
  Demux/2 -> magneSensor1/1(In1)
  Demux/1 -> magneSensor/1(In1)
  atitude/1 -> Demux/1
  magneSensor/1(Out1) -> Mux/1  "x"
  magneSensor1/1(Out1) -> Mux/2  "y"
  magneSensor2/1(Out1) -> Mux/3  "z"
  Mux/1 -> atitudeSen/1

== system SFF_Simulator/Atuadores de Atitude/Atuador atitude ativado/Magnetorquer ativado/Magnetômetro/If Action Subsystem1 ==
  atitude : Inport
  Action Port : ActionPort  ActionPortLabel=else
  atitudeSen : Outport
  wires:
  atitude/1 -> atitudeSen/1

== system SFF_Simulator/Atuadores de Atitude/Atuador atitude ativado/Magnetorquer ativado/Magnetômetro/If Action Subsystem/magneSensor ==
  In1 : Inport
  Add1 : Sum
  Add2 : Sum
  Constant : Constant  Value=magne_bias
  Random Source1 : dspsrcs4/Random Source  SrcType=Uniform  MinVal=-magne_ruido  MaxVal=magne_ruido  MeanVal=0  VarVal=1  RepMode=Not repeatable  rawSeed=1  IsInherit=off  SampTime=step_modelo  SampFrame=1  OutComplex=Real  DataType=double  SimulateUsing=Code generation
  Out1 : Outport
  wires:
  Random Source1/1 -> Add2/1
  In1/1 -> Add1/2
  Constant/1 -> Add1/1
  Add1/1 -> Add2/2
  Add2/1 -> Out1/1

== system SFF_Simulator/Atuadores de Atitude/Atuador atitude ativado/Magnetorquer ativado/Magnetômetro/If Action Subsystem/magneSensor1 ==
  In1 : Inport
  Add1 : Sum
  Add2 : Sum
  Constant : Constant  Value=magne_bias
  Random Source1 : dspsrcs4/Random Source  SrcType=Uniform  MinVal=-magne_ruido  MaxVal=magne_ruido  MeanVal=0  VarVal=1  RepMode=Not repeatable  rawSeed=1  IsInherit=off  SampTime=step_modelo  SampFrame=1  OutComplex=Real  DataType=double  SimulateUsing=Code generation
  Out1 : Outport
  wires:
  Add2/1 -> Out1/1
  Add1/1 -> Add2/2
  Random Source1/1 -> Add2/1
  In1/1 -> Add1/2
  Constant/1 -> Add1/1

== system SFF_Simulator/Atuadores de Atitude/Atuador atitude ativado/Magnetorquer ativado/Magnetômetro/If Action Subsystem/magneSensor2 ==
  In1 : Inport
  Add1 : Sum
  Add2 : Sum
  Constant : Constant  Value=magne_bias
  Random Source1 : dspsrcs4/Random Source  SrcType=Uniform  MinVal=-magne_ruido  MaxVal=magne_ruido  MeanVal=0  VarVal=1  RepMode=Not repeatable  rawSeed=1  IsInherit=off  SampTime=step_modelo  SampFrame=1  OutComplex=Real  DataType=double  SimulateUsing=Code generation
  Out1 : Outport
  wires:
  Add2/1 -> Out1/1
  Add1/1 -> Add2/2
  Random Source1/1 -> Add2/1
  In1/1 -> Add1/2
  Constant/1 -> Add1/1

== matlab function SFF_Simulator/Atuadores Orbital/acelSistLVLHSeg1 ==
  data: A_q input; acelx output; m1 input; F_b input; acely output; acelz output
function [acelx,acely,acelz] = fcn(A_q,m1,F_b)

F_real = A_q'*F_b;

Fx_real = F_real(1);
Fy_real = F_real(2);
Fz_real = F_real(3);


acelx = Fx_real/m1;
acely = Fy_real/m1;
acelz = Fz_real/m1;

== matlab function SFF_Simulator/Atuadores Orbital/forçasSistCorpoSeg ==
  data: A_q input; Fx_b output; m1 input; controleOrbital input; Fy_b output; Fz_b output
function [Fx_b,Fy_b,Fz_b] = fcn(A_q,m1,controleOrbital)

ux = controleOrbital(1);
uy = controleOrbital(2);
uz = controleOrbital(3);

Fx = m1*ux;
Fy = m1*uy;
Fz = m1*uz;

F_b = A_q*[Fx; Fy; Fz];

Fx_b = F_b(1);
Fy_b = F_b(2);
Fz_b = F_b(3);

== matlab function SFF_Simulator/Atuadores de Atitude/Atuador atitude ativado/Magnetorquer ativado/Conjunto Rodas de Reação + Magnetotorques/B_matriz ==
  data: B_seg input; y output
function y = fcn(B_seg)

Bx = B_seg(1);
By = B_seg(2);
Bz = B_seg(3);

y = [0 0 -By
    -Bz 1 Bx
    By 0 0];

== matlab function SFF_Simulator/Atuadores de Atitude/Atuador atitude ativado/Magnetorquer ativado/Conjunto Rodas de Reação + Magnetotorques/Inv_B_matriz ==
  data: B_seg input; y output
function y = fcn(B_seg)

Bx = B_seg(1);
By = B_seg(2);
Bz = B_seg(3);

if By == 0
    y = [0 0 0; 0 0 0; 0 0 0];
else
    y = (1/(By^2))*[0 0 By
    Bx*By By^2 By*Bz
    -By 0 0];
end

== matlab function SFF_Simulator/Dinâmica Cinemática Atitude/MATLAB Function ==
  data: u input; phi output; theta output; psi output
function [phi,theta,psi] = fcn(u)

y = quat2eul([u(4) u(1) u(2) u(3)]);

phi = wrapToPi(y(1));
theta = wrapToPi(y(2));
psi = wrapToPi(y(3));
